simulink model "MASc_AndriyPredmyrskyy_SAC"  (R2020a)
settings: Solver=FixedStepAuto  StartTime=0.0  StopTime=tsim  FixedStep=baseRate  RelTol=1e-3  EnableMultiTasking=on
values from neighbouring files (symbols this model uses):
  Amp1off = 0.2    [Run_Initializer.m]
  Amp2off = 0.1    [Run_Initializer.m]
  baseRate = 0.05    [Run_Initializer.m]
  BLACKMass = 12.3341    [LoadResults.m]    (also in Run_Initializer.m = model_param(3))
  Cmout = [eye(3,3),zeros(3,3)]    [Run_Initializer.m]    (also in SimpleSAC.m = [alpha*eye(3,3),eye(3,3)])
  D = 0    [OptimizationPlots.m]    (also in OptimizeSAC_DE.m; OptimizeSAC_DE_CHANGE.m; OptimizeSAC_PSO.m; SADE_OptimizationForSAC.m)
  drop_states_BLACK = [2.3,1.5,0.176047682762146]    [Run_Initializer.m]
  drop_states_BLUE = [ xLength/2+0.9; yLength/2+0.5; 0]    [Run_Initializer.m]
  drop_states_RED = [2.60644311523438,1.21791186523438,3.08142089843750]    [Run_Initializer.m]
  F_thrusters_BLACK = 0.25.*ones(8,1)    [Run_Initializer.m]
  F_thrusters_BLUE = 0.25.*ones(8,1)    [Run_Initializer.m]
  F_thrusters_RED = 0.25.*ones(8,1)    [Run_Initializer.m]
  GeI = X(2,Best_i).*eye(3)    [OptimizeSAC_DE.m]    (also in OptimizeSAC_DE_CHANGE.m; OptimizeSAC_PSO.m = pos(besti,5).*eye(3); RunAllOptimizations.m = Init.GeI; SADE_OptimizationForSAC.m)
  GeP = X(1,Best_i).*eye(3)    [OptimizeSAC_DE.m]    (also in OptimizeSAC_DE_CHANGE.m; OptimizeSAC_PSO.m = pos(besti,1).*eye(3); RunAllOptimizations.m = Init.GeP; SADE_OptimizationForSAC.m)
  GuI = X(4,Best_i).*eye(3)    [OptimizeSAC_DE.m]    (also in OptimizeSAC_DE_CHANGE.m; OptimizeSAC_PSO.m = pos(besti,8).*eye(3); RunAllOptimizations.m = Init.GuI; SADE_OptimizationForSAC.m)
  GuP = X(3,Best_i).*eye(3)    [OptimizeSAC_DE.m]    (also in OptimizeSAC_DE_CHANGE.m; OptimizeSAC_PSO.m = pos(besti,4).*eye(3); RunAllOptimizations.m = Init.GuP; SADE_OptimizationForSAC.m)
  GxI = blkdiag(X(7,Best_i).*eye(3),X(8,Best_i).*eye(3))    [OptimizeSAC_DE.m]    (also in OptimizeSAC_DE_CHANGE.m = X(6,Best_i).*eye(6); OptimizeSAC_PSO.m = blkdiag(pos(besti,6).*eye(3),pos(besti,7).*eye(3)); RunAllOptimizations.m = Init.GxI; SADE_OptimizationForSAC.m)
  GxP = blkdiag(X(5,Best_i).*eye(3),X(6,Best_i).*eye(3))    [OptimizeSAC_DE.m]    (also in OptimizeSAC_DE_CHANGE.m = X(5,Best_i).*eye(6); OptimizeSAC_PSO.m = blkdiag(pos(besti,2).*eye(3),pos(besti,3).*eye(3)); RunAllOptimizations.m = Init.GxP; SADE_OptimizationForSAC.m)
  GzI = 1e0.*eye(12)    [Run_Initializer.m]
  GzP = 0e-2.*eye(12)    [Run_Initializer.m]
  home_states_BLACK = LastPosition    [Run_Initializer.m]
  home_states_BLUE = [ xLength/2-0.9; yLength/2+0.5; 0]    [Run_Initializer.m]
  home_states_RED = [ xLength/2+0.7; yLength/2; 0]    [Run_Initializer.m]
  init_states_BLACK = FirstPosition    [Run_Initializer.m]
  init_states_BLUE = [ xLength/2+0.9; yLength/2+0.5; 0]    [Run_Initializer.m]
  init_states_RED = [ xLength/2+0.7; yLength/2; 0]    [Run_Initializer.m]
  K = 3    [Run_Initializer.m]    (also in cycloid.m)
  K_Force = 1    [Run_Initializer.m]
  Kd_Force = 3    [Run_Initializer.m]
  Kd_tb = 0.4    [Run_Initializer.m]
  Kd_tblue = 0.4    [Run_Initializer.m]
  Kd_tr = 0.4    [Run_Initializer.m]
  Kd_xb = 5    [Run_Initializer.m]
  Kd_xblue = 5    [Run_Initializer.m]
  Kd_xr = 5    [Run_Initializer.m]
  Kd_yb = 5    [Run_Initializer.m]
  Kd_yblue = 5    [Run_Initializer.m]
  Kd_yr = 5    [Run_Initializer.m]
  KeI0 = 0.*[   0.1063   -0.0058         0 ... (first row only)    [Run_Initializer.m]    (also in SimpleSAC.m = zeros(3))
  Kp_tb = 0.1    [Run_Initializer.m]
  Kp_tblue = 0.1    [Run_Initializer.m]
  Kp_tr = 0.1    [Run_Initializer.m]
  Kp_xb = 2    [Run_Initializer.m]
  Kp_xblue = 2    [Run_Initializer.m]
  Kp_xr = 2    [Run_Initializer.m]
  Kp_yb = 2    [Run_Initializer.m]
  Kp_yblue = 2    [Run_Initializer.m]
  Kp_yr = 2    [Run_Initializer.m]
  KuI0 = 0.*0.2193*[1,0,0;0,1,0;0,0,0]    [Run_Initializer.m]    (also in SimpleSAC.m = zeros(3))
  KxI0 = 0.*[-0.2193*eye(3),-3.2891*eye(3)]    [Run_Initializer.m]    (also in SimpleSAC.m = zeros(3,6))
  KzI0 = zeros(3,12)    [Run_Initializer.m]
  noise_variance_BLACK = 0    [Run_Initializer.m]
  noise_variance_BLUE = 0    [Run_Initializer.m]
  noise_variance_RED = 0    [Run_Initializer.m]
  omega = 0.03    [LoadResults.m]    (also in OptimizeSAC_PSO.m = 0.2; Run_Initializer.m = 0.06; SPSO_OptimizationForSAC.m = 0.2; SimpleSAC.m = sqrt(Force./(Mass*Radius)))
  omega1off = 0.03    [Run_Initializer.m]
  omega2off = 0.06    [Run_Initializer.m]
  Phase0_End = Phase0_Duration    (= 10)    [Run_Initializer.m]
  Phase1_End = Phase0_Duration + Phase1_Duration    (= 15)    [Run_Initializer.m]
  phase1off = 2*pi + 3-2+1.0654    (= 8.34858530718)    [Run_Initializer.m]
  Phase2_End = Phase0_Duration + Phase1_Duration +                                   Phase2_Duration    (= 35)    [Run_Initializer.m]
  phase2off = mod(pi^66,2*pi)    [Run_Initializer.m]
  Phase3_End = Phase0_Duration + Phase1_Duration +                                   Phase2_Duration + Phase3_Duration    (= 246)    [Run_Initializer.m]
  Phase3_SubPhase1_End = Phase2_End + Phase3_SubPhase1_Duration    (= 40)    [Run_Initializer.m]
  Phase3_SubPhase2_End = Phase2_End + Phase3_SubPhase1_Duration +                                   Phase3_SubPhase2_Duration    (= 45)    [Run_Initializer.m]
  Phase3_SubPhase3_End = Phase2_End + Phase3_SubPhase1_Duration +                                   Phase3_SubPhase2_Duration +                                  Phase3_SubPhase3_Duration    (= 46)    [Run_Initializer.m]
  Phase3_SubPhase4_End = Phase2_End + Phase3_SubPhase1_Duration +                                   Phase3_SubPhase2_Duration +                                  Phase3_SubPhase3_Duration +                                  Phase3_SubPhase4_Duration    [Run_Initializer.m]
  Phase4_End = Phase0_Duration + Phase1_Duration +                                   Phase2_Duration + Phase3_Duration +                                   Phase4_Duration    (= 266)    [Run_Initializer.m]
  Phase5_End = Phase0_Duration + Phase1_Duration +                                   Phase2_Duration + Phase3_Duration +                                   Phase4_Duration + Phase5_Duration    (= 271)    [Run_Initializer.m]
  platformSelection = 1    [OptimizationPlots.m]    (also in OptimizeSAC_DE.m; OptimizeSAC_DE_CHANGE.m; OptimizeSAC_PSO.m; SADE_OptimizationForSAC.m)
  serverRate = 0.1    [Run_Initializer.m]    (also in SimpleSAC.m)
  sigma_eI = X(9,Best_i)    [OptimizeSAC_DE.m]    (also in OptimizeSAC_DE_CHANGE.m = X(7,Best_i); OptimizeSAC_PSO.m = pos(besti,9); RunAllOptimizations.m = Init.sigma_eI; SADE_OptimizationForSAC.m)
  sigma_uI = X(10,Best_i)    [OptimizeSAC_DE.m]    (also in OptimizeSAC_DE_CHANGE.m = X(8,Best_i); OptimizeSAC_PSO.m = pos(besti,11); RunAllOptimizations.m = Init.sigma_uI; SADE_OptimizationForSAC.m)
  sigma_xI = X(11,Best_i)    [OptimizeSAC_DE.m]    (also in OptimizeSAC_DE_CHANGE.m = X(9,Best_i); OptimizeSAC_PSO.m = pos(besti,10); RunAllOptimizations.m = Init.sigma_xI; SADE_OptimizationForSAC.m)
  sigma_zI = 0    [Run_Initializer.m]
  sysd1 = c2d(sys,baseRate,opt)    [Run_Initializer.m]    (also in SimpleSAC.m = c2d(sys,serverRate,opt))
  sysd2 = c2d(sysInverse,baseRate,opt)    [Run_Initializer.m]
  thruster_dist2CG_BLACK = [83.42;-52.58;55.94;-60.05;54.08;-53.92;77.06;-55.94]    [Run_Initializer.m]
  thruster_dist2CG_BLUE = [83.42;-52.58;55.94;-60.05;54.08;-53.92;77.06;-55.94]    [Run_Initializer.m]
  thruster_dist2CG_RED = [49.92;-78.08;70.46;-63.54;81.08;-50.42;57.44;-75.96]    [Run_Initializer.m]
  xm2_ini = -(sysd2.D(1,1).*xm_ini(1:3))./(sysd2.C(1,1))    [Run_Initializer.m]
  xm_ini = [FirstPosition(1), FirstPosition(2), 0, 0, 0, 0]'    [Run_Initializer.m]    (also in SimpleSAC.m = [0, 0, 0, 0, 0, 0]')
undefined symbols (not defined in the file or in its folder): DiscIntNeverNeededParam, G3, simMode, WhoAmI
libraries: dspstat3 x18, simulink x12, raspberrypiBasiclib x10, dspsigops x9, embdlinuxlib x8, mspfiltlib x3, dsparch4 x3, peGeneralControl x3, eeGeneralControl x3, dspswit3 x2, MainLibrary x2, sensehatlib x1
(part 10 of 11)

== system MASc_AndriyPredmyrskyy_SAC/Phase #3: Experiment/Change BLACK Behavior/Sub-Phase #4/Adaptive Control/Subsystem3/anti-Saturation Flag ==
  Before Signal : Inport
  After Signal : Inport  Port=2
  Demux : Demux  Outputs=3
  Demux1 : Demux  Outputs=3
  NOT : Subsystem
  OR : Subsystem
  OR1 : Subsystem
  Saturation Detection Flag1 : Subsystem
  Saturation Detection Flag2 : Subsystem
  Saturation Detection Flag3 : Subsystem
  Out1 : Outport  VectorParamsAs1DForOutWhenUnconnected=off
  wires:
  NOT/1(Out1) -> Out1/1
  Before Signal/1 -> Demux/1
  Demux/1 -> Saturation Detection Flag1/1(Before Signal)
  After Signal/1 -> Demux1/1
  Demux1/1 -> Saturation Detection Flag1/2(After Signal)
  Demux1/2 -> Saturation Detection Flag2/2(After Signal)
  Demux/2 -> Saturation Detection Flag2/1(Before Signal)
  Demux/3 -> Saturation Detection Flag3/1(Before Signal)
  Demux1/3 -> Saturation Detection Flag3/2(After Signal)
  OR/1(Out1) -> OR1/1(In1)
  Saturation Detection Flag1/1(Out1) -> OR/1(In1)
  Saturation Detection Flag2/1(Out1) -> OR/2(In2)
  Saturation Detection Flag3/1(Out1) -> OR1/2(In2)
  OR1/1(Out1) -> NOT/1(In1)

== system MASc_AndriyPredmyrskyy_SAC/Phase #3: Experiment/Change BLACK Behavior/Sub-Phase #4/Adaptive Control/Subsystem5/DAC SAC ==
  Model Reference Error : Inport
  Disturbance Model : Inport  Port=2
  Constant : Constant  Value=GzI
  Constant1 : Constant  Value=GzP
  Discrete-Time Integrator5 : DiscreteIntegrator  InitialCondition=KzI0  SampleTime=-1  ICPrevOutput=DiscIntNeverNeededParam  ICPrevScaledInput=DiscIntNeverNeededParam
  Gain : Gain  Gain=sigma_zI
  Matrix Multiply : Product  Inputs=3  Multiplication=Matrix(*)
  Matrix Multiply1 : Product  Inputs=3  Multiplication=Matrix(*)
  Matrix Multiply2 : Product  Multiplication=Matrix(*)
  Mux : Mux  Inputs=3
  Reshape : Reshape  OutputDimensionality=Column vector (2-D)  OutputDimensions=[4,3]
  Reshape3 : Reshape
  Reshape4 : Reshape
  Reshape5 : Reshape
  Scope : Scope
  Scope1 : Scope
  Scope2 : Scope
  Sum : Sum  Inputs=|++
  Sum1 : Sum  Inputs=|+-
  To Workspace1 : ToWorkspace  VariableName=SACKz  SaveFormat=Timeseries  SampleTime=-1
  Transpose : Math  Operator=transpose  SignedPower=on  SaturateOnIntegerOverflow=on
  Output Force : Outport  VectorParamsAs1DForOutWhenUnconnected=off
  wires:
  Disturbance Model/1 -> Scope1/1, Matrix Multiply2/2, Transpose/1
  Matrix Multiply1/1 -> Sum/1
  Matrix Multiply/1 -> Sum1/1
  Transpose/1 -> Matrix Multiply1/2, Matrix Multiply/2
  Sum/1 -> Scope/1, Reshape3/1, Matrix Multiply2/1
  Reshape/1 -> Matrix Multiply1/1, Matrix Multiply/1
  Constant1/1 -> Matrix Multiply1/3
  Discrete-Time Integrator5/1 -> Sum/2, Reshape4/1, Gain/1
  Matrix Multiply2/1 -> Output Force/1, Scope2/1
  Sum1/1 -> Reshape5/1, Discrete-Time Integrator5/1
  Gain/1 -> Sum1/2
  Model Reference Error/1 -> Reshape/1
  Constant/1 -> Matrix Multiply/3
  Mux/1 -> To Workspace1/1
  Reshape3/1 -> Mux/1
  Reshape4/1 -> Mux/2
  Reshape5/1 -> Mux/3

== system MASc_AndriyPredmyrskyy_SAC/Phase #3: Experiment/Change BLACK Behavior/Sub-Phase #4/Adaptive Control/Subsystem5/Disturbance Generator1 ==
  Positional Disturbance Generator : Subsystem
  Scope2 : Scope
  Disturbance Model Output : Outport  VectorParamsAs1DForOutWhenUnconnected=off
  wires:
  Positional Disturbance Generator/1(Out1) -> Scope2/1, Disturbance Model Output/1

== system MASc_AndriyPredmyrskyy_SAC/Phase #3: Experiment/Change BLACK Behavior/Sub-Phase #4/Adaptive Control/Subsystem5/Subsystem ==
  In1 : Inport
  Demux : Demux  Outputs=3
  Demux1 : Demux  Outputs=3
  Discrete Derivative : simulink/Discrete/Discrete Derivative  gainval=1.0  ICPrevScaledInput=0.0  OutMin=[]  OutMax=[]  OutDataType=fixdt(1, 16)  OutScaling=2^-10  DoSatur=off
  Mux : Mux  Inputs=12
  Out1 : Outport  VectorParamsAs1DForOutWhenUnconnected=off
  wires:
  In1/1 -> Demux/1, Discrete Derivative/1
  Demux/1 -> Mux/3, Mux/1
  Demux/2 -> Mux/7, Mux/5
  Demux/3 -> Mux/11, Mux/9
  Discrete Derivative/1 -> Demux1/1
  Demux1/1 -> Mux/4, Mux/2
  Demux1/2 -> Mux/8, Mux/6
  Demux1/3 -> Mux/12, Mux/10
  Mux/1 -> Out1/1

== system MASc_AndriyPredmyrskyy_SAC/Phase #3: Experiment/Change BLACK Behavior/Sub-Phase #4/Adaptive Control/Subsystem5/Subsystem1 ==
  In1 : Inport
  Demux : Demux  Outputs=3
  Demux1 : Demux  Outputs=3
  Discrete-Time Integrator : DiscreteIntegrator  SampleTime=-1  ICPrevOutput=DiscIntNeverNeededParam  ICPrevScaledInput=DiscIntNeverNeededParam
  Discrete-Time Integrator1 : DiscreteIntegrator  SampleTime=-1  ICPrevOutput=DiscIntNeverNeededParam  ICPrevScaledInput=DiscIntNeverNeededParam
  Gain : Gain  Gain=-1./100
  Mux : Mux  Inputs=12
  Out1 : Outport  VectorParamsAs1DForOutWhenUnconnected=off
  wires:
  Demux/1 -> Mux/3, Mux/1
  Demux/2 -> Mux/7, Mux/5
  Demux/3 -> Mux/11, Mux/9
  Demux1/1 -> Mux/4, Mux/2
  Demux1/2 -> Mux/8, Mux/6
  Demux1/3 -> Mux/12, Mux/10
  Mux/1 -> Out1/1
  In1/1 -> Gain/1
  Discrete-Time Integrator/1 -> Demux1/1, Discrete-Time Integrator1/1
  Discrete-Time Integrator1/1 -> Demux/1
  Gain/1 -> Discrete-Time Integrator/1

== system MASc_AndriyPredmyrskyy_SAC/Phase #3: Experiment/Change BLACK Behavior/Sub-Phase #4/Custom Discrete PD (Attitude)/x_dot -> x1/Hold this value ==
  In1 : Inport
  Action Port : ActionPort
  Out1 : Outport  VectorParamsAs1DForOutWhenUnconnected=off
  wires:
  In1/1 -> Out1/1

== system MASc_AndriyPredmyrskyy_SAC/Phase #3: Experiment/Change BLACK Behavior/Sub-Phase #4/LQR/Discrete Derivative/Subsystem ==
  note: dy/dt ~= (y2-y1)/deltaT
  x : Inport
  Delay1 : Delay  DelayLength=1  InitialConditionSource=Input port
      settings: InputPortMap=u0,p4
  Hold this value : Subsystem  TreatAsAtomicUnit=on
  Sum6 : Sum  Inputs=-+|
  divide by delta T : Gain  Gain=1/serverRate
  "if we went through a \"step\"" : If  IfExpression=u1 ~= 0  ShowElse=off
  dx/dt : Outport  VectorParamsAs1DForOutWhenUnconnected=off
  wires:
  Delay1/1 -> Sum6/1
  divide by delta T/1 -> dx/dt/1
  "if we went through a \"step\""/1 -> Hold this value/Action
  x/1 -> Sum6/2, Delay1/2, Delay1/1
  Hold this value/1(Out1) -> divide by delta T/1
  Sum6/1 -> "if we went through a \"step\""/1, Hold this value/1(In1)

== system MASc_AndriyPredmyrskyy_SAC/Phase #3: Experiment/Change BLACK Behavior/Sub-Phase #4/LQR/Discrete Derivative/Subsystem1 ==
  note: dy/dt ~= (y2-y1)/deltaT
  y : Inport
  Delay1 : Delay  DelayLength=1  InitialConditionSource=Input port
      settings: InputPortMap=u0,p4
  Hold this value : Subsystem  TreatAsAtomicUnit=on
  Sum6 : Sum  Inputs=-+|
  divide by delta T : Gain  Gain=1/serverRate
  "if we went through a \"step\"" : If  IfExpression=u1 ~= 0  ShowElse=off
  dy/dt : Outport  VectorParamsAs1DForOutWhenUnconnected=off
  wires:
  Delay1/1 -> Sum6/1
  divide by delta T/1 -> dy/dt/1
  "if we went through a \"step\""/1 -> Hold this value/Action
  y/1 -> Sum6/2, Delay1/2, Delay1/1
  Hold this value/1(Out1) -> divide by delta T/1
  Sum6/1 -> "if we went through a \"step\""/1, Hold this value/1(In1)

== system MASc_AndriyPredmyrskyy_SAC/Phase #3: Experiment/Change BLACK Behavior/Sub-Phase #4/LQR/Discrete Derivative/Subsystem2 ==
  note: dy/dt ~= (y2-y1)/deltaT
  z : Inport
  Delay1 : Delay  DelayLength=1  InitialConditionSource=Input port
      settings: InputPortMap=u0,p4
  Hold this value : Subsystem  TreatAsAtomicUnit=on
  Sum6 : Sum  Inputs=-+|
  divide by delta T : Gain  Gain=1/serverRate
  "if we went through a \"step\"" : If  IfExpression=u1 ~= 0  ShowElse=off
  dy/dt : Outport  VectorParamsAs1DForOutWhenUnconnected=off
  wires:
  Delay1/1 -> Sum6/1
  divide by delta T/1 -> dy/dt/1
  "if we went through a \"step\""/1 -> Hold this value/Action
  z/1 -> Sum6/2, Delay1/2, Delay1/1
  Hold this value/1(Out1) -> divide by delta T/1
  Sum6/1 -> "if we went through a \"step\""/1, Hold this value/1(In1)

== system MASc_AndriyPredmyrskyy_SAC/Phase #3: Experiment/Change BLUE Behavior/Sub-Phase #1/Custom Discrete PD (Attitude)/x_dot -> x1/Hold this value ==
  In1 : Inport
  Action Port : ActionPort
  Out1 : Outport  VectorParamsAs1DForOutWhenUnconnected=off
  wires:
  In1/1 -> Out1/1

== system MASc_AndriyPredmyrskyy_SAC/Phase #3: Experiment/Change BLUE Behavior/Sub-Phase #1/Custom Discrete PD (X-Position)/x_dot -> x1/Hold this value ==
  In1 : Inport
  Action Port : ActionPort
  Out1 : Outport  VectorParamsAs1DForOutWhenUnconnected=off
  wires:
  In1/1 -> Out1/1

== system MASc_AndriyPredmyrskyy_SAC/Phase #3: Experiment/Change BLUE Behavior/Sub-Phase #1/Custom Discrete PD (Y-Position)/x_dot -> x1/Hold this value ==
  In1 : Inport
  Action Port : ActionPort
  Out1 : Outport  VectorParamsAs1DForOutWhenUnconnected=off
  wires:
  In1/1 -> Out1/1

== system MASc_AndriyPredmyrskyy_SAC/Phase #3: Experiment/Change BLUE Behavior/Sub-Phase #4/Custom Discrete PD (Attitude)/x_dot -> x1/Hold this value ==
  In1 : Inport
  Action Port : ActionPort
  Out1 : Outport  VectorParamsAs1DForOutWhenUnconnected=off
  wires:
  In1/1 -> Out1/1

== system MASc_AndriyPredmyrskyy_SAC/Phase #3: Experiment/Change BLUE Behavior/Sub-Phase #4/Custom Discrete PD (X-Position)/x_dot -> x1/Hold this value ==
  In1 : Inport
  Action Port : ActionPort
  Out1 : Outport  VectorParamsAs1DForOutWhenUnconnected=off
  wires:
  In1/1 -> Out1/1

== system MASc_AndriyPredmyrskyy_SAC/Phase #3: Experiment/Change BLUE Behavior/Sub-Phase #4/Custom Discrete PD (Y-Position)/x_dot -> x1/Hold this value ==
  In1 : Inport
  Action Port : ActionPort
  Out1 : Outport  VectorParamsAs1DForOutWhenUnconnected=off
  wires:
  In1/1 -> Out1/1

== system MASc_AndriyPredmyrskyy_SAC/Phase #3: Experiment/Change RED Behavior/Sub-Phase #1/Custom Discrete PD (Attitude)/x_dot -> x1/Hold this value ==
  In1 : Inport
  Action Port : ActionPort
  Out1 : Outport  VectorParamsAs1DForOutWhenUnconnected=off
  wires:
  In1/1 -> Out1/1

== system MASc_AndriyPredmyrskyy_SAC/Phase #3: Experiment/Change RED Behavior/Sub-Phase #1/Custom Discrete PD (X-Position)/x_dot -> x1/Hold this value ==
  In1 : Inport
  Action Port : ActionPort
  Out1 : Outport  VectorParamsAs1DForOutWhenUnconnected=off
  wires:
  In1/1 -> Out1/1

== system MASc_AndriyPredmyrskyy_SAC/Phase #3: Experiment/Change RED Behavior/Sub-Phase #1/Custom Discrete PD (Y-Position)/x_dot -> x1/Hold this value ==
  In1 : Inport
  Action Port : ActionPort
  Out1 : Outport  VectorParamsAs1DForOutWhenUnconnected=off
  wires:
  In1/1 -> Out1/1

== system MASc_AndriyPredmyrskyy_SAC/Phase #3: Experiment/Change RED Behavior/Sub-Phase #4/Custom Discrete PD (Attitude)/x_dot -> x1/Hold this value ==
  In1 : Inport
  Action Port : ActionPort
  Out1 : Outport  VectorParamsAs1DForOutWhenUnconnected=off
  wires:
  In1/1 -> Out1/1

== system MASc_AndriyPredmyrskyy_SAC/Phase #3: Experiment/Change RED Behavior/Sub-Phase #4/Custom Discrete PD (X-Position)/x_dot -> x1/Hold this value ==
  In1 : Inport
  Action Port : ActionPort
  Out1 : Outport  VectorParamsAs1DForOutWhenUnconnected=off
  wires:
  In1/1 -> Out1/1

== system MASc_AndriyPredmyrskyy_SAC/Phase #3: Experiment/Change RED Behavior/Sub-Phase #4/Custom Discrete PD (Y-Position)/x_dot -> x1/Hold this value ==
  In1 : Inport
  Action Port : ActionPort
  Out1 : Outport  VectorParamsAs1DForOutWhenUnconnected=off
  wires:
  In1/1 -> Out1/1

== system MASc_AndriyPredmyrskyy_SAC/Phase #3: Experiment/Change BLACK Behavior/Sub-Phase #4/Adaptive Control/Subsystem3/anti-Saturation Flag/NOT ==
  In1 : Inport
  Constant : Constant
  Gain : Gain  Gain=-1
  Sum : Sum  Inputs=|++
  Out1 : Outport  VectorParamsAs1DForOutWhenUnconnected=off
  wires:
  In1/1 -> Gain/1
  Gain/1 -> Sum/1
  Sum/1 -> Out1/1
  Constant/1 -> Sum/2

== system MASc_AndriyPredmyrskyy_SAC/Phase #3: Experiment/Change BLACK Behavior/Sub-Phase #4/Adaptive Control/Subsystem3/anti-Saturation Flag/OR ==
  In1 : Inport
  In2 : Inport  Port=2
  Saturation : Saturate  UpperLimit=1
  Sum3 : Sum  Inputs=|++
  Out1 : Outport  VectorParamsAs1DForOutWhenUnconnected=off
  wires:
  Sum3/1 -> Saturation/1
  In2/1 -> Sum3/2
  Saturation/1 -> Out1/1
  In1/1 -> Sum3/1

== system MASc_AndriyPredmyrskyy_SAC/Phase #3: Experiment/Change BLACK Behavior/Sub-Phase #4/Adaptive Control/Subsystem3/anti-Saturation Flag/OR1 ==
  In1 : Inport
  In2 : Inport  Port=2
  Saturation : Saturate  UpperLimit=1
  Sum3 : Sum  Inputs=|++
  Out1 : Outport  VectorParamsAs1DForOutWhenUnconnected=off
  wires:
  Sum3/1 -> Saturation/1
  In2/1 -> Sum3/2
  Saturation/1 -> Out1/1
  In1/1 -> Sum3/1

== system MASc_AndriyPredmyrskyy_SAC/Phase #3: Experiment/Change BLACK Behavior/Sub-Phase #4/Adaptive Control/Subsystem3/anti-Saturation Flag/Saturation Detection Flag1 ==
  Before Signal : Inport
  After Signal : Inport  Port=2
  Abs : Abs
  Constant : Constant  Value=0
  Constant1 : Constant
  Sum : Sum  Inputs=|+-
  Switch : Switch  Criteria=u2 > Threshold
  Out1 : Outport  VectorParamsAs1DForOutWhenUnconnected=off
  wires:
  Before Signal/1 -> Sum/2
  Constant1/1 -> Switch/1
  Constant/1 -> Switch/3
  Sum/1 -> Abs/1
  Abs/1 -> Switch/2
  Switch/1 -> Out1/1
  After Signal/1 -> Sum/1

== system MASc_AndriyPredmyrskyy_SAC/Phase #3: Experiment/Change BLACK Behavior/Sub-Phase #4/Adaptive Control/Subsystem3/anti-Saturation Flag/Saturation Detection Flag2 ==
  Before Signal : Inport
  After Signal : Inport  Port=2
  Abs : Abs
  Constant : Constant  Value=0
  Constant1 : Constant
  Sum : Sum  Inputs=|+-
  Switch : Switch  Criteria=u2 > Threshold
  Out1 : Outport  VectorParamsAs1DForOutWhenUnconnected=off
  wires:
  Before Signal/1 -> Sum/2
  Constant1/1 -> Switch/1
  Constant/1 -> Switch/3
  Sum/1 -> Abs/1
  Abs/1 -> Switch/2
  Switch/1 -> Out1/1
  After Signal/1 -> Sum/1

== system MASc_AndriyPredmyrskyy_SAC/Phase #3: Experiment/Change BLACK Behavior/Sub-Phase #4/Adaptive Control/Subsystem3/anti-Saturation Flag/Saturation Detection Flag3 ==
  Before Signal : Inport
  After Signal : Inport  Port=2
  Abs : Abs
  Constant : Constant  Value=0
  Constant1 : Constant
  Sum : Sum  Inputs=|+-
  Switch : Switch  Criteria=u2 > Threshold
  Out1 : Outport  VectorParamsAs1DForOutWhenUnconnected=off
  wires:
  Before Signal/1 -> Sum/2
  Constant1/1 -> Switch/1
  Constant/1 -> Switch/3
  Sum/1 -> Abs/1
  Abs/1 -> Switch/2
  Switch/1 -> Out1/1
  After Signal/1 -> Sum/1

== system MASc_AndriyPredmyrskyy_SAC/Phase #3: Experiment/Change BLACK Behavior/Sub-Phase #4/Adaptive Control/Subsystem5/Disturbance Generator1/Positional Disturbance Generator ==
  Constant : Constant  Value=0
  Constant1 : Constant  Value=0
  Mux{,1,3..4} (4 alike) : Mux
  Mux2 : Mux  Inputs=3
  Mux5 : Mux  Inputs=2
  Mux6 : Mux  Inputs=2
  Sine Wave : Sin  Frequency=omega1off  SampleTime=0
  Sine Wave1 : Sin  Amplitude=omega1off  Frequency=omega1off  Phase=pi/2  SampleTime=0
  Sine Wave10 : Sin  Frequency=omega*K  SampleTime=0
  Sine Wave11 : Sin  Frequency=omega*K  Phase=pi/2  SampleTime=0
  Sine Wave2 : Sin  Frequency=omega1off  Phase=pi/2  SampleTime=0
  Sine Wave3 : Sin  Amplitude=omega1off  Frequency=omega1off  Phase=pi  SampleTime=0
  Sine Wave4 : Sin  Frequency=omega2off  SampleTime=0
  Sine Wave5 : Sin  Amplitude=omega2off  Frequency=omega2off  Phase=pi/2  SampleTime=0
  Sine Wave6 : Sin  Frequency=omega2off  Phase=pi/2  SampleTime=0
  Sine Wave7 : Sin  Amplitude=omega2off  Frequency=omega2off  Phase=pi  SampleTime=0
  Sine Wave8 : Sin  Frequency=omega  SampleTime=0
  Sine Wave9 : Sin  Frequency=omega  Phase=pi/2  SampleTime=0
  Out1 : Outport  VectorParamsAs1DForOutWhenUnconnected=off
  wires:
  Sine Wave/1 -> Mux/1
  Sine Wave1/1 -> Mux/2
  Sine Wave2/1 -> Mux/3
  Sine Wave3/1 -> Mux/4
  Sine Wave6/1 -> Mux1/3
  Sine Wave4/1 -> Mux1/1
  Sine Wave5/1 -> Mux1/2
  Sine Wave7/1 -> Mux1/4
  Mux/1 -> Mux2/1
  Mux1/1 -> Mux2/2
  Mux3/1 -> Mux2/3
  Constant/1 -> Mux3/4, Mux3/3, Mux3/2, Mux3/1
  Mux5/1 -> Mux6/2
  Constant1/1 -> Mux5/1, Mux5/2
  Mux4/1 -> Mux6/1
  Sine Wave10/1 -> Mux4/2
  Sine Wave8/1 -> Mux4/1
  Sine Wave9/1 -> Mux4/3
  Sine Wave11/1 -> Mux4/4
  Mux2/1 -> Out1/1

== system MASc_AndriyPredmyrskyy_SAC/Phase #3: Experiment/Change BLACK Behavior/Sub-Phase #4/LQR/Discrete Derivative/Subsystem/Hold this value ==
  In1 : Inport
  Action Port : ActionPort
  Out1 : Outport  VectorParamsAs1DForOutWhenUnconnected=off
  wires:
  In1/1 -> Out1/1

== system MASc_AndriyPredmyrskyy_SAC/Phase #3: Experiment/Change BLACK Behavior/Sub-Phase #4/LQR/Discrete Derivative/Subsystem1/Hold this value ==
  In1 : Inport
  Action Port : ActionPort
  Out1 : Outport  VectorParamsAs1DForOutWhenUnconnected=off
  wires:
  In1/1 -> Out1/1

== system MASc_AndriyPredmyrskyy_SAC/Phase #3: Experiment/Change BLACK Behavior/Sub-Phase #4/LQR/Discrete Derivative/Subsystem2/Hold this value ==
  In1 : Inport
  Action Port : ActionPort
  Out1 : Outport  VectorParamsAs1DForOutWhenUnconnected=off
  wires:
  In1/1 -> Out1/1

== matlab function MASc_AndriyPredmyrskyy_SAC/Phase #2: Move to Initial Position/Change BLACK Behavior/Hough Control/MATLAB Function3 ==
  data: z input; Ox output
function Ox    = C3( z )
%C3 gives the rotation matrix about the z-axis for an angle 'z'
%   z - the angle about the z-axis which you rotate
%   A - the rotation matrix

Ox = [cos(z) sin(z); -sin(z) cos(z)]*[1;0];
end

== matlab function MASc_AndriyPredmyrskyy_SAC/Phase #2: Move to Initial Position/Change BLACK Behavior/Hough Control/MATLAB Function4 ==
  data: Oy input; e_out output; e_in input
function e_out = fcn(Oy, e_in)

a = sign(Oy'*e_in);
e_out = -a*norm(e_in);

== matlab function MASc_AndriyPredmyrskyy_SAC/From Force//Torque to PWM Signal/Change BLACK Behavior/Calculate Thruster ON//OFF/MATLAB Function ==
  data: H output; thruster_dist2CG_BLACK parameter; F_thrusters_BLACK parameter
function H = MakeH(thruster_dist2CG_BLACK,F_thrusters_BLACK)

Vec1 = [ -1
         -1
          0 
          0
          1
          1
          0
          0 ];
      
Vec2 = [  0
          0
          1
          1
          0
          0
         -1
         -1 ];
     
Vec3 = thruster_dist2CG_BLACK./1000;

Mat1 = [Vec1, Vec2, Vec3]';

Mat2 = diag((F_thrusters_BLACK./2));

H    = Mat1*Mat2;

end

== matlab function MASc_AndriyPredmyrskyy_SAC/Phase #3: Experiment/Change BLACK Behavior/Sub-Phase #4/BLACK_RzD/Wrap1/MATLAB Function ==
  data: u input; wrappedAngle output
function wrappedAngle = wrapAngle(u)

wrappedAngle = atan2(sin(u),cos(u));

end

== matlab function MASc_AndriyPredmyrskyy_SAC/Phase #3: Experiment/Change BLACK Behavior/Sub-Phase #4/Adaptive Control/Simple Adaptive Controller/Subsystem/MATLAB Function ==
  data: um input; u output; xm input; ey input; KeI input; KxI input; KuI input; Ke output; Kx output; Ku output; KeI_dot output; KxI_dot output; KuI_dot output; GeP parameter; GxP parameter; GuP parameter; GeI parameter; GxI parameter; GuI parameter; sigma_eI parameter; sigma_xI parameter; sigma_uI parameter
function [u, Ke, Kx, Ku, KeI_dot, KxI_dot, KuI_dot]  = AdaptionLaw(um, xm,...
    ey, KeI, KxI, KuI, GeP, GxP, GuP, GeI, GxI, GuI, sigma_eI, sigma_xI,...
sigma_uI)

Kep = ey*transpose(ey)*GeP;
Kxp = ey*transpose(xm)*GxP;
Kup = ey*transpose(um)*GuP;

Ke = Kep+KeI;
Kx = Kxp+KxI;
Ku = Kup+KuI;

KeI_dot = ey*transpose(ey)*GeI - sigma_eI*KeI;
KxI_dot = ey*transpose(xm)*GxI - KxI*sigma_xI;%This is the only way the sizes make sense...
KuI_dot = ey*transpose(um)*GuI - sigma_uI*KuI;

u  = Ke*ey + Kx*xm + Ku*um;

end

== matlab function MASc_AndriyPredmyrskyy_SAC/From Force//Torque to PWM Signal/Change BLACK Behavior/Calculate Thruster ON//OFF/MATLAB Function1 ==
  data: H output; thruster_dist2CG_BLACK parameter; F_thrusters_BLACK parameter
function H = MakeH(thruster_dist2CG_BLACK,F_thrusters_BLACK)

Vec1 = [ -1
         -1
          0 
          0
          1
          1
          0
          0 ];
      
Vec2 = [  0
          0
          1
          1
          0
          0
         -1
         -1 ];
     
Vec3 = thruster_dist2CG_BLACK./1000;

Mat1 = [Vec1, Vec2, Vec3]';

Mat2 = diag((F_thrusters_BLACK));

H    = Mat1*Mat2;

end

== matlab function MASc_AndriyPredmyrskyy_SAC/From Force//Torque to PWM Signal/Change BLACK Behavior/Calculate Thruster ON//OFF/MATLAB Function2 ==
  data: ThrustPer_Final output; ThrustPer input
function ThrustPer_Final  = ThrusterSat(ThrustPer)

ValveTime       = 0.007;
TControl        = 0.1;
ThrustPer_Final = zeros(8,1);

if max(ThrustPer) > 1
    ThrustPer_Sat = ThrustPer/max(ThrustPer);
else
    ThrustPer_Sat = ThrustPer;
end

for i = 1:8
    if ThrustPer_Sat(i) > ValveTime/TControl 
        ThrustPer_Final(i) = ThrustPer_Sat(i);
    else
        ThrustPer_Final(i) = 0;
    end
end
   

end

== matlab function MASc_AndriyPredmyrskyy_SAC/From Force//Torque to PWM Signal/Change BLACK Behavior/Calculate Thruster ON//OFF/Rotate Forces to Inertial/Create Rotation Matrix ==
  data: Rz input; C_Ib output
function C_Ib = RotateFrame(Rz)

C_bI = [  cos(Rz) sin(Rz)
         -sin(Rz) cos(Rz) ];

C_Ib = inv(C_bI);

end

== matlab function MASc_AndriyPredmyrskyy_SAC/From Force//Torque to PWM Signal/Change BLACK Behavior/Rotate Forces to Body/Create Rotation Matrix ==
  data: Rz input; C_bI output
function C_bI = RotateFrame(Rz)

C_bI = [  cos(Rz) sin(Rz)
         -sin(Rz) cos(Rz) ];

end

== matlab function MASc_AndriyPredmyrskyy_SAC/From Force//Torque to PWM Signal/Change RED Behavior/Calculate Thruster ON//OFF/MATLAB Function ==
  data: H output; thruster_dist2CG_RED parameter; F_thrusters_RED parameter
function H = MakeH(thruster_dist2CG_RED,F_thrusters_RED)

Vec1 = [ -1
         -1
          0 
          0
          1
          1
          0
          0 ];
      
Vec2 = [  0
          0
          1
          1
          0
          0
         -1
         -1 ];
     
Vec3 = thruster_dist2CG_RED./1000;

Mat1 = [Vec1, Vec2, Vec3]';

Mat2 = diag((F_thrusters_RED./2));

H    = Mat1*Mat2;

end

== matlab function MASc_AndriyPredmyrskyy_SAC/From Force//Torque to PWM Signal/Change RED Behavior/Calculate Thruster ON//OFF/MATLAB Function1 ==
  data: H output; thruster_dist2CG_RED parameter; F_thrusters_RED parameter
function H = MakeH(thruster_dist2CG_RED,F_thrusters_RED)

Vec1 = [ -1
         -1
          0 
          0
          1
          1
          0
          0 ];
      
Vec2 = [  0
          0
          1
          1
          0
          0
         -1
         -1 ];
     
Vec3 = thruster_dist2CG_RED./1000;

Mat1 = [Vec1, Vec2, Vec3]';

Mat2 = diag((F_thrusters_RED));

H    = Mat1*Mat2;

end

== matlab function MASc_AndriyPredmyrskyy_SAC/From Force//Torque to PWM Signal/Change RED Behavior/Calculate Thruster ON//OFF/MATLAB Function2 ==
  data: ThrustPer_Final output; ThrustPer input
function ThrustPer_Final  = ThrusterSat(ThrustPer)

ValveTime       = 0.007;
TControl        = 0.1;
ThrustPer_Final = zeros(8,1);

if max(ThrustPer) > 1
    ThrustPer_Sat = ThrustPer/max(ThrustPer);
else
    ThrustPer_Sat = ThrustPer;
end

for i = 1:8
    if ThrustPer_Sat(i) > ValveTime/TControl 
        ThrustPer_Final(i) = ThrustPer_Sat(i);
    else
        ThrustPer_Final(i) = 0;
    end
end
   

end

== matlab function MASc_AndriyPredmyrskyy_SAC/From Force//Torque to PWM Signal/Change RED Behavior/Calculate Thruster ON//OFF/Rotate Forces to Inertial/Create Rotation Matrix ==
  data: Rz input; C_Ib output
function C_Ib = RotateFrame(Rz)

C_bI = [  cos(Rz) sin(Rz)
         -sin(Rz) cos(Rz) ];

C_Ib = inv(C_bI);

end

== matlab function MASc_AndriyPredmyrskyy_SAC/Simulate Plant Dynamics/Sample and Hold Data to Match PhaseSpace (RED)/MATLAB Function ==
  data: TIME input; y output; SERVER input
function y = fcn(TIME, SERVER)

if mod(TIME,SERVER) == 0
    y = 1;
else
    y = 0;
end

== matlab function MASc_AndriyPredmyrskyy_SAC/Simulate Plant Dynamics/Sample and Hold Data to Match PhaseSpace (BLACK)/MATLAB Function ==
  data: TIME input; y output; SERVER input
function y = fcn(TIME, SERVER)

if mod(TIME,SERVER) == 0
    y = 1;
else
    y = 0;
end

== matlab function MASc_AndriyPredmyrskyy_SAC/From Force//Torque to PWM Signal/Change RED Behavior/Rotate Forces to Body/Create Rotation Matrix ==
  data: Rz input; C_bI output
function C_bI = RotateFrame(Rz)

C_bI = [  cos(Rz) sin(Rz)
         -sin(Rz) cos(Rz) ];

end

== matlab function MASc_AndriyPredmyrskyy_SAC/Phase #2: Move to Initial Position/Change RED Behavior/Hough Control/MATLAB Function2 ==
  data: Oy output; z input; Ox output
function [Oy, Ox]   = C3( z )
%C3 gives the rotation matrix about the z-axis for an angle 'z'
%   z - the angle about the z-axis which you rotate
%   A - the rotation matrix

Ox = [cos(z) sin(z); -sin(z) cos(z)]*[1;0];
Oy = [cos(z) sin(z); -sin(z) cos(z)]*[0;1];
end

== matlab function MASc_AndriyPredmyrskyy_SAC/Phase #2: Move to Initial Position/Change RED Behavior/Hough Control/MATLAB Function3 ==
  data: z input; Ox output
function Ox    = C3( z )
%C3 gives the rotation matrix about the z-axis for an angle 'z'
%   z - the angle about the z-axis which you rotate
%   A - the rotation matrix

Ox = [cos(z) sin(z); -sin(z) cos(z)]*[1;0];
end

== matlab function MASc_AndriyPredmyrskyy_SAC/Phase #2: Move to Initial Position/Change RED Behavior/Hough Control/MATLAB Function4 ==
  data: Oy input; e_out output; e_in input
function e_out = fcn(Oy, e_in)

a = sign(Oy'*e_in);
e_out = -a*norm(e_in);

== matlab function MASc_AndriyPredmyrskyy_SAC/Phase #3: Experiment/Change BLACK Behavior/Sub-Phase #4/Hough Control/MATLAB Function2 ==
  data: Oy output; z input; Ox output
function [Oy, Ox]   = C3( z )
%C3 gives the rotation matrix about the z-axis for an angle 'z'
%   z - the angle about the z-axis which you rotate
%   A - the rotation matrix

Ox = [cos(z) sin(z); -sin(z) cos(z)]*[1;0];
Oy = [cos(z) sin(z); -sin(z) cos(z)]*[0;1];
end

== matlab function MASc_AndriyPredmyrskyy_SAC/Simulate Plant Dynamics/BLUE  Dynamics Model/MATLAB Function ==
  data: control_inputs input; x_ddot output; model_param parameter
function x_ddot = BLUE_dynamics(control_inputs, model_param)

%#codegen
% Fully define the size of x_ddot() for code generation:
x_ddot     = zeros(3,1);

% Extract the servicer model parameters from the model_param vector defined
% in initialize.m:
m_BLUE    = model_param(5);
I_BLUE    = model_param(6);

% Extract the control inputs from the control_input vector:
Fx        = control_inputs(1);              % [N]
Fy        = control_inputs(2);              % [N]
Tz        = control_inputs(3);              % [N.m]

% Calculate the state acceleration vector:
x_ddot(1) = Fx/m_BLUE;                      % [m/s^2]
x_ddot(2) = Fy/m_BLUE;                      % [m/s^2]
x_ddot(3) = Tz/I_BLUE;                      % [rad/s^2]

end

== matlab function MASc_AndriyPredmyrskyy_SAC/Phase #4: Return Home/Change BLACK Behavior/Hough Control/MATLAB Function2 ==
  data: Oy output; z input; Ox output
function [Oy, Ox]   = C3( z )
%C3 gives the rotation matrix about the z-axis for an angle 'z'
%   z - the angle about the z-axis which you rotate
%   A - the rotation matrix

Ox = [cos(z) sin(z); -sin(z) cos(z)]*[1;0];
Oy = [cos(z) sin(z); -sin(z) cos(z)]*[0;1];
end

== matlab function MASc_AndriyPredmyrskyy_SAC/Phase #4: Return Home/Change BLACK Behavior/Hough Control/MATLAB Function3 ==
  data: z input; Ox output
function Ox    = C3( z )
%C3 gives the rotation matrix about the z-axis for an angle 'z'
%   z - the angle about the z-axis which you rotate
%   A - the rotation matrix

Ox = [cos(z) sin(z); -sin(z) cos(z)]*[1;0];
end

== matlab function MASc_AndriyPredmyrskyy_SAC/Phase #4: Return Home/Change BLACK Behavior/Hough Control/MATLAB Function4 ==
  data: Oy input; e_out output; e_in input
function e_out = fcn(Oy, e_in)

a = sign(Oy'*e_in);
e_out = -a*norm(e_in);

== matlab function MASc_AndriyPredmyrskyy_SAC/Phase #4: Return Home/Change RED Behavior/Hough Control/MATLAB Function2 ==
  data: Oy output; z input; Ox output
function [Oy, Ox]   = C3( z )
%C3 gives the rotation matrix about the z-axis for an angle 'z'
%   z - the angle about the z-axis which you rotate
%   A - the rotation matrix

Ox = [cos(z) sin(z); -sin(z) cos(z)]*[1;0];
Oy = [cos(z) sin(z); -sin(z) cos(z)]*[0;1];
end

== matlab function MASc_AndriyPredmyrskyy_SAC/Phase #4: Return Home/Change RED Behavior/Hough Control/MATLAB Function3 ==
  data: z input; Ox output
function Ox    = C3( z )
%C3 gives the rotation matrix about the z-axis for an angle 'z'
%   z - the angle about the z-axis which you rotate
%   A - the rotation matrix

Ox = [cos(z) sin(z); -sin(z) cos(z)]*[1;0];
end

== matlab function MASc_AndriyPredmyrskyy_SAC/Phase #4: Return Home/Change RED Behavior/Hough Control/MATLAB Function4 ==
  data: Oy input; e_out output; e_in input
function e_out = fcn(Oy, e_in)

a = sign(Oy'*e_in);
e_out = -a*norm(e_in);

== matlab function MASc_AndriyPredmyrskyy_SAC/Phase #2: Move to Initial Position/Change BLUE Behavior/Hough Control/MATLAB Function2 ==
  data: Oy output; z input; Ox output
function [Oy, Ox]   = C3( z )
%C3 gives the rotation matrix about the z-axis for an angle 'z'
%   z - the angle about the z-axis which you rotate
%   A - the rotation matrix

Ox = [cos(z) sin(z); -sin(z) cos(z)]*[1;0];
Oy = [cos(z) sin(z); -sin(z) cos(z)]*[0;1];
end

== matlab function MASc_AndriyPredmyrskyy_SAC/Phase #2: Move to Initial Position/Change BLUE Behavior/Hough Control/MATLAB Function3 ==
  data: z input; Ox output
function Ox    = C3( z )
%C3 gives the rotation matrix about the z-axis for an angle 'z'
%   z - the angle about the z-axis which you rotate
%   A - the rotation matrix

Ox = [cos(z) sin(z); -sin(z) cos(z)]*[1;0];
end

== matlab function MASc_AndriyPredmyrskyy_SAC/Phase #2: Move to Initial Position/Change BLUE Behavior/Hough Control/MATLAB Function4 ==
  data: Oy input; e_out output; e_in input
function e_out = fcn(Oy, e_in)

a = sign(Oy'*e_in);
e_out = -a*norm(e_in);

== matlab function MASc_AndriyPredmyrskyy_SAC/Phase #3: Experiment/Change BLUE Behavior/Sub-Phase #1/Hough Control/MATLAB Function2 ==
  data: Oy output; z input; Ox output
function [Oy, Ox]   = C3( z )
%C3 gives the rotation matrix about the z-axis for an angle 'z'
%   z - the angle about the z-axis which you rotate
%   A - the rotation matrix

Ox = [cos(z) sin(z); -sin(z) cos(z)]*[1;0];
Oy = [cos(z) sin(z); -sin(z) cos(z)]*[0;1];
end

== matlab function MASc_AndriyPredmyrskyy_SAC/Simulate Plant Dynamics/RED Dynamics Model/MATLAB Function ==
  data: control_inputs input; x_ddot output; model_param parameter
function x_ddot = RED_dynamics(control_inputs, model_param)

%#codegen
% Fully define the size of x_ddot() for code generation:
x_ddot     = zeros(3,1);

% Extract the servicer model parameters from the model_param vector defined
% in initialize.m:
m_RED    = model_param(1);
I_RED    = model_param(2);

% Extract the control inputs from the control_input vector:
Fx        = control_inputs(1);              % [N]
Fy        = control_inputs(2);              % [N]
Tz        = control_inputs(3);              % [N.m]

% Calculate the state acceleration vector:
x_ddot(1) = Fx/m_RED;                      % [m/s^2]
x_ddot(2) = Fy/m_RED;                      % [m/s^2]
x_ddot(3) = Tz/I_RED;                      % [rad/s^2]

end

== matlab function MASc_AndriyPredmyrskyy_SAC/Phase #3: Experiment/Change RED Behavior/Sub-Phase #1/Hough Control/MATLAB Function2 ==
  data: Oy output; z input; Ox output
function [Oy, Ox]   = C3( z )
%C3 gives the rotation matrix about the z-axis for an angle 'z'
%   z - the angle about the z-axis which you rotate
%   A - the rotation matrix

Ox = [cos(z) sin(z); -sin(z) cos(z)]*[1;0];
Oy = [cos(z) sin(z); -sin(z) cos(z)]*[0;1];
end

== matlab function MASc_AndriyPredmyrskyy_SAC/Phase #3: Experiment/Change RED Behavior/Sub-Phase #1/Hough Control/MATLAB Function3 ==
  data: z input; Ox output
function Ox    = C3( z )
%C3 gives the rotation matrix about the z-axis for an angle 'z'
%   z - the angle about the z-axis which you rotate
%   A - the rotation matrix

Ox = [cos(z) sin(z); -sin(z) cos(z)]*[1;0];
end

== matlab function MASc_AndriyPredmyrskyy_SAC/Phase #3: Experiment/Change RED Behavior/Sub-Phase #1/Hough Control/MATLAB Function4 ==
  data: Oy input; e_out output; e_in input
function e_out = fcn(Oy, e_in)

a = sign(Oy'*e_in);
e_out = -a*norm(e_in);

== matlab function MASc_AndriyPredmyrskyy_SAC/Phase #3: Experiment/Change BLUE Behavior/Sub-Phase #1/Hough Control/MATLAB Function3 ==
  data: z input; Ox output
function Ox    = C3( z )
%C3 gives the rotation matrix about the z-axis for an angle 'z'
%   z - the angle about the z-axis which you rotate
%   A - the rotation matrix

Ox = [cos(z) sin(z); -sin(z) cos(z)]*[1;0];
end

== matlab function MASc_AndriyPredmyrskyy_SAC/Phase #3: Experiment/Change BLUE Behavior/Sub-Phase #1/Hough Control/MATLAB Function4 ==
  data: Oy input; e_out output; e_in input
function e_out = fcn(Oy, e_in)

a = sign(Oy'*e_in);
e_out = -a*norm(e_in);

== matlab function MASc_AndriyPredmyrskyy_SAC/Phase #3: Experiment/Change BLUE Behavior/Sub-Phase #4/Hough Control/MATLAB Function2 ==
  data: Oy output; z input; Ox output
function [Oy, Ox]   = C3( z )
%C3 gives the rotation matrix about the z-axis for an angle 'z'
%   z - the angle about the z-axis which you rotate
%   A - the rotation matrix

Ox = [cos(z) sin(z); -sin(z) cos(z)]*[1;0];
Oy = [cos(z) sin(z); -sin(z) cos(z)]*[0;1];
end

== matlab function MASc_AndriyPredmyrskyy_SAC/Phase #3: Experiment/Change RED Behavior/Sub-Phase #4/Hough Control/MATLAB Function2 ==
  data: Oy output; z input; Ox output
function [Oy, Ox]   = C3( z )
%C3 gives the rotation matrix about the z-axis for an angle 'z'
%   z - the angle about the z-axis which you rotate
%   A - the rotation matrix

Ox = [cos(z) sin(z); -sin(z) cos(z)]*[1;0];
Oy = [cos(z) sin(z); -sin(z) cos(z)]*[0;1];
end

== matlab function MASc_AndriyPredmyrskyy_SAC/Phase #3: Experiment/Change RED Behavior/Sub-Phase #4/Hough Control/MATLAB Function3 ==
  data: z input; Ox output
function Ox    = C3( z )
%C3 gives the rotation matrix about the z-axis for an angle 'z'
%   z - the angle about the z-axis which you rotate
%   A - the rotation matrix

Ox = [cos(z) sin(z); -sin(z) cos(z)]*[1;0];
end

== matlab function MASc_AndriyPredmyrskyy_SAC/Phase #3: Experiment/Change RED Behavior/Sub-Phase #4/Hough Control/MATLAB Function4 ==
  data: Oy input; e_out output; e_in input
function e_out = fcn(Oy, e_in)

a = sign(Oy'*e_in);
e_out = -a*norm(e_in);

== matlab function MASc_AndriyPredmyrskyy_SAC/Phase #3: Experiment/Change BLACK Behavior/Sub-Phase #4/Hough Control/MATLAB Function3 ==
  data: z input; Ox output
function Ox    = C3( z )
%C3 gives the rotation matrix about the z-axis for an angle 'z'
%   z - the angle about the z-axis which you rotate
%   A - the rotation matrix

Ox = [cos(z) sin(z); -sin(z) cos(z)]*[1;0];
end

== matlab function MASc_AndriyPredmyrskyy_SAC/Phase #3: Experiment/Change BLACK Behavior/Sub-Phase #1/Hough Control/MATLAB Function2 ==
  data: Oy output; z input; Ox output
function [Oy, Ox]   = C3( z )
%C3 gives the rotation matrix about the z-axis for an angle 'z'
%   z - the angle about the z-axis which you rotate
%   A - the rotation matrix

Ox = [cos(z) sin(z); -sin(z) cos(z)]*[1;0];
Oy = [cos(z) sin(z); -sin(z) cos(z)]*[0;1];
end

== matlab function MASc_AndriyPredmyrskyy_SAC/Simulate Plant Dynamics/BLACK Dynamics Model/MATLAB Function ==
  data: control_inputs input; x_ddot output; model_param parameter
function x_ddot = BLACK_dynamics(control_inputs, model_param)

%#codegen
% Fully define the size of x_ddot() for code generation:
x_ddot     = zeros(3,1);

% Extract the servicer model parameters from the model_param vector defined
% in initialize.m:
m_BLACK    = model_param(3);
I_BLACK    = model_param(4);

% Extract the control inputs from the control_input vector:
Fx        = control_inputs(1);              % [N]
Fy        = control_inputs(2);              % [N]
Tz        = control_inputs(3);              % [N.m]

% Calculate the state acceleration vector:
x_ddot(1) = Fx/m_BLACK;                      % [m/s^2]
x_ddot(2) = Fy/m_BLACK;                      % [m/s^2]
x_ddot(3) = Tz/I_BLACK;                      % [rad/s^2]

end

== matlab function MASc_AndriyPredmyrskyy_SAC/Phase #3: Experiment/Change BLACK Behavior/Sub-Phase #1/Hough Control/MATLAB Function3 ==
  data: z input; Ox output
function Ox    = C3( z )
%C3 gives the rotation matrix about the z-axis for an angle 'z'
%   z - the angle about the z-axis which you rotate
%   A - the rotation matrix

Ox = [cos(z) sin(z); -sin(z) cos(z)]*[1;0];
end

== matlab function MASc_AndriyPredmyrskyy_SAC/Phase #3: Experiment/Change BLACK Behavior/Sub-Phase #1/Hough Control/MATLAB Function4 ==
  data: Oy input; e_out output; e_in input
function e_out = fcn(Oy, e_in)

a = sign(Oy'*e_in);
e_out = -a*norm(e_in);

== matlab function MASc_AndriyPredmyrskyy_SAC/Phase #3: Experiment/Change BLUE Behavior/Sub-Phase #4/Hough Control/MATLAB Function3 ==
  data: z input; Ox output
function Ox    = C3( z )
%C3 gives the rotation matrix about the z-axis for an angle 'z'
%   z - the angle about the z-axis which you rotate
%   A - the rotation matrix

Ox = [cos(z) sin(z); -sin(z) cos(z)]*[1;0];
end

== matlab function MASc_AndriyPredmyrskyy_SAC/Phase #3: Experiment/Change BLUE Behavior/Sub-Phase #4/Hough Control/MATLAB Function4 ==
  data: Oy input; e_out output; e_in input
function e_out = fcn(Oy, e_in)

a = sign(Oy'*e_in);
e_out = -a*norm(e_in);

== matlab function MASc_AndriyPredmyrskyy_SAC/Phase #5: Hold Home/Change BLACK Behavior/Hough Control/MATLAB Function2 ==
  data: Oy output; z input; Ox output
function [Oy, Ox]   = C3( z )
%C3 gives the rotation matrix about the z-axis for an angle 'z'
%   z - the angle about the z-axis which you rotate
%   A - the rotation matrix

Ox = [cos(z) sin(z); -sin(z) cos(z)]*[1;0];
Oy = [cos(z) sin(z); -sin(z) cos(z)]*[0;1];
end

== matlab function MASc_AndriyPredmyrskyy_SAC/Phase #5: Hold Home/Change BLACK Behavior/Hough Control/MATLAB Function3 ==
  data: z input; Ox output
function Ox    = C3( z )
%C3 gives the rotation matrix about the z-axis for an angle 'z'
%   z - the angle about the z-axis which you rotate
%   A - the rotation matrix

Ox = [cos(z) sin(z); -sin(z) cos(z)]*[1;0];
end

== matlab function MASc_AndriyPredmyrskyy_SAC/Phase #5: Hold Home/Change BLACK Behavior/Hough Control/MATLAB Function4 ==
  data: Oy input; e_out output; e_in input
function e_out = fcn(Oy, e_in)

a = sign(Oy'*e_in);
e_out = -a*norm(e_in);

== matlab function MASc_AndriyPredmyrskyy_SAC/Phase #4: Return Home/Change BLUE Behavior/Hough Control/MATLAB Function2 ==
  data: Oy output; z input; Ox output
function [Oy, Ox]   = C3( z )
%C3 gives the rotation matrix about the z-axis for an angle 'z'
%   z - the angle about the z-axis which you rotate
%   A - the rotation matrix

Ox = [cos(z) sin(z); -sin(z) cos(z)]*[1;0];
Oy = [cos(z) sin(z); -sin(z) cos(z)]*[0;1];
end

== matlab function MASc_AndriyPredmyrskyy_SAC/Phase #4: Return Home/Change BLUE Behavior/Hough Control/MATLAB Function3 ==
  data: z input; Ox output
function Ox    = C3( z )
%C3 gives the rotation matrix about the z-axis for an angle 'z'
%   z - the angle about the z-axis which you rotate
%   A - the rotation matrix

Ox = [cos(z) sin(z); -sin(z) cos(z)]*[1;0];
end

== matlab function MASc_AndriyPredmyrskyy_SAC/Phase #4: Return Home/Change BLUE Behavior/Hough Control/MATLAB Function4 ==
  data: Oy input; e_out output; e_in input
function e_out = fcn(Oy, e_in)

a = sign(Oy'*e_in);
e_out = -a*norm(e_in);

== matlab function MASc_AndriyPredmyrskyy_SAC/Simulate Plant Dynamics/Sample and Hold Data to Match PhaseSpace (BLUE)/MATLAB Function ==
  data: TIME input; y output; SERVER input
function y = fcn(TIME, SERVER)

if mod(TIME,SERVER) == 0
    y = 1;
else
    y = 0;
end

== matlab function MASc_AndriyPredmyrskyy_SAC/Phase #5: Hold Home/Change RED Behavior/Hough Control/MATLAB Function2 ==
  data: Oy output; z input; Ox output
function [Oy, Ox]   = C3( z )
%C3 gives the rotation matrix about the z-axis for an angle 'z'
%   z - the angle about the z-axis which you rotate
%   A - the rotation matrix

Ox = [cos(z) sin(z); -sin(z) cos(z)]*[1;0];
Oy = [cos(z) sin(z); -sin(z) cos(z)]*[0;1];
end

== matlab function MASc_AndriyPredmyrskyy_SAC/Phase #5: Hold Home/Change RED Behavior/Hough Control/MATLAB Function3 ==
  data: z input; Ox output
function Ox    = C3( z )
%C3 gives the rotation matrix about the z-axis for an angle 'z'
%   z - the angle about the z-axis which you rotate
%   A - the rotation matrix

Ox = [cos(z) sin(z); -sin(z) cos(z)]*[1;0];
end

== matlab function MASc_AndriyPredmyrskyy_SAC/Phase #5: Hold Home/Change RED Behavior/Hough Control/MATLAB Function4 ==
  data: Oy input; e_out output; e_in input
function e_out = fcn(Oy, e_in)

a = sign(Oy'*e_in);
e_out = -a*norm(e_in);

== matlab function MASc_AndriyPredmyrskyy_SAC/Phase #5: Hold Home/Change BLUE Behavior/Hough Control/MATLAB Function2 ==
  data: Oy output; z input; Ox output
function [Oy, Ox]   = C3( z )
%C3 gives the rotation matrix about the z-axis for an angle 'z'
%   z - the angle about the z-axis which you rotate
%   A - the rotation matrix

Ox = [cos(z) sin(z); -sin(z) cos(z)]*[1;0];
Oy = [cos(z) sin(z); -sin(z) cos(z)]*[0;1];
end

== matlab function MASc_AndriyPredmyrskyy_SAC/Phase #5: Hold Home/Change BLUE Behavior/Hough Control/MATLAB Function3 ==
  data: z input; Ox output
function Ox    = C3( z )
%C3 gives the rotation matrix about the z-axis for an angle 'z'
%   z - the angle about the z-axis which you rotate
%   A - the rotation matrix

Ox = [cos(z) sin(z); -sin(z) cos(z)]*[1;0];
end

== matlab function MASc_AndriyPredmyrskyy_SAC/Phase #5: Hold Home/Change BLUE Behavior/Hough Control/MATLAB Function4 ==
  data: Oy input; e_out output; e_in input
function e_out = fcn(Oy, e_in)

a = sign(Oy'*e_in);
e_out = -a*norm(e_in);
